simulink model "Pruefungsaufgabe_15"  (R2017b)
settings: Solver=ode45  StartTime=0.0  StopTime=5  FixedStep=0.001  MaxStep=1e-3  RelTol=1e-3  EnableMultiTasking=on
values from neighbouring files (symbols this model uses):
  CR = 2    [Pruefungsaufgabe_15_Konstanten.m]
  JRED = m1*R^2/(Ue^2*WGrad)    (= 0.000444444444444)    [Pruefungsaufgabe_15_Konstanten.m]
  KM = 38.4E-3    (= 0.0384)    [Pruefungsaufgabe_10_Konstanten.m]    (also in Pruefungsaufgabe_13_Konstanten.m = 0.05; Pruefungsaufgabe_15_Konstanten.m = 0.05)
  R = 0.02    [Pruefungsaufgabe_15_Konstanten.m]
  RA = 4.99    [Pruefungsaufgabe_10_Konstanten.m]    (also in Pruefungsaufgabe_13_Konstanten.m = 0.6; Pruefungsaufgabe_15_Konstanten.m = 5)
  Ue = 2    [Pruefungsaufgabe_15_Konstanten.m]
  WGrad = 0.9    [Pruefungsaufgabe_15_Konstanten.m]
undefined symbols (not defined in the file or in its folder): sigbuilder_block
libraries: simulink x2
settings Model: Creator=jbaur  LastModifiedBy=jbaur
settings DataIOCC: ExternalInput=X1  SaveFormat=StructureWithTime  InspectSignalLogs=on  SignalLoggingName=sigsOut
settings OptimizationCC: DefaultParameterBehavior=Inlined  InlineInvariantSignals=on  BufferReuse=off  ExpressionDepthLimit=2147483647  InitFltsAndDblsToZero=on  LifeSpan=inf
settings DebuggingCC: SaveWithParameterizedLinksMsg=none  SignalResolutionControl=TryResolveAllWithWarning  MultiTaskDSMMsg=warning  MultiTaskCondExecSysMsg=none  StateNameClashWarn=warning  InitInArrayFormatMsg=none  SFUnexpectedBacktrackingDiag=warning  SFNoUnconditionalDefaultTransitionDiag=warning  SFExecutionAtInitializationDiag=none
settings HardwareCC: ProdBitPerPointer=32  ProdBitPerSizeT=32  ProdBitPerPtrDiffT=32  ProdLargestAtomicFloat=None  ProdIntDivRoundTo=Undefined  ProdEndianess=Unspecified  ProdWordSize=32  ProdHWDeviceType=32-bit Generic  TargetBitPerPointer=64  TargetBitPerSizeT=64  TargetBitPerPtrDiffT=64  TargetLongLongMode=on  TargetIntDivRoundTo=Zero  TargetEndianess=LittleEndian  TargetWordSize=64  TargetHWDeviceType=MATLAB Host  ProdEqTarget=off
settings ModelReferenceCC: PropagateSignalLabelsOutOfModel=off
settings CodeAppCC: StateflowObjectComments=on
settings GRTTargetCC: TargetFcnLib=ansi_tfl_tmw.mat  TargetLangStandard=C89/C90 (ANSI)  ModelReferenceCompliant=off  GeneratePreprocessorConditionals=Disable all  CombineOutputUpdateFcns=off  MatFileLogging=off  GRTInterface=on
settings ConfigComp: CovMetricSettings=dw  CovHtmlReporting=on  CovSaveCumulativeToWorkspaceVar=on  CovSaveSingleToWorkspaceVar=on  CovExternalEMLEnable=off  CovSFcnEnable=off

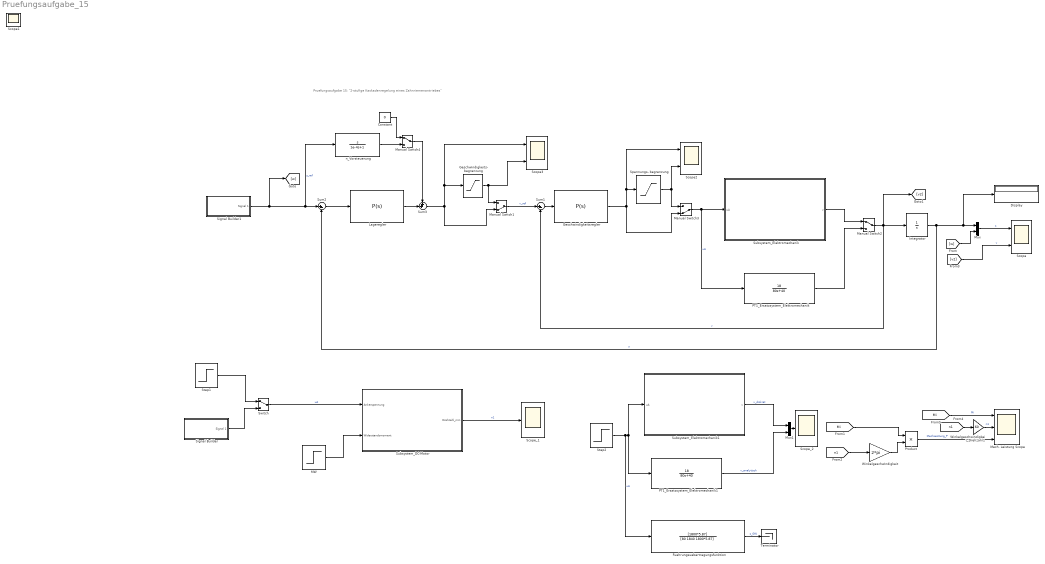
== system Pruefungsaufgabe_15 ==
  note: Pruefungsaufgabe 15: "2-stufige Kaskadenregelung eines Zahnriemenantriebes"
  Constant : Constant  Value=0
  Display : Display
  Fuehrungsuebertragungsfunktion : TransferFcn  Numerator=[1800*5.87]  Denominator=[80 1840 1800*5.87]
  Geschwindigkeits- begrenzung : Saturate  UpperLimit=4.77  LowerLimit=-4.77
  Geschwindigkeitsregler : simulink/Continuous/PID Controller  Controller=P  TimeDomain=Continuous-time  SampleTime=-1  IntegratorMethod=Forward Euler  FilterMethod=Forward Euler  Form=Parallel  UseFilter=on  ControllerParametersSource=internal  P=100  I=1000  D=0  N=1000  InitialConditionSource=internal  InitialConditionForIntegrator=0  InitialConditionForFilter=0  ExternalReset=none  LimitOutput=off  UpperSaturationLimit=24  LowerSaturationLimit=-24  LinearizeAsGain=off  AntiWindupMode=clamping  Kb=1000  TrackingMode=off  Kt=1  PParamMin=[]  PParamMax=[]  IParamMin=[]  IParamMax=[]  DParamMin=[]  DParamMax=[]  NParamMin=[]  NParamMax=[]  KbParamMin=[]  KbParamMax=[]  KtParamMin=[]  KtParamMax=[]  POutMin=[]  POutMax=[]  IOutMin=[]  IOutMax=[]  DOutMin=[]  DOutMax=[]  NOutMin=[]  NOutMax=[]  KbOutMin=[]  KbOutMax=[]  KtOutMin=[]  KtOutMax=[]  IntegratorOutMin=[]  IntegratorOutMax=[]  FilterOutMin=[]  FilterOutMax=[]  SumOutMin=[]  SumOutMax=[]  SumI1OutMin=[]  SumI1OutMax=[]  SumI2OutMin=[]  SumI2OutMax=[]  SumI3OutMin=[]  SumI3OutMax=[]  SumDOutMin=[]  SumDOutMax=[]  SaturationOutMin=[]  SaturationOutMax=[]  IntegratorContinuousStateAttributes=''  IntegratorStateMustResolveToSignalObject=off  IntegratorRTWStateStorageClass=Auto  FilterContinuousStateAttributes=''  FilterStateMustResolveToSignalObject=off  FilterRTWStateStorageClass=Auto  DifferentiatorICPrevScaledInput=0  DifferentiatorOutMin=[]  DifferentiatorOutMax=[]  InitialConditionSetting=State (most efficient)  FilterDiffOutCoefMin=[]  FilterDiffOutCoefMax=[]  SumDenOutMin=[]  SumDenOutMax=[]  SumNumOutMin=[]  SumNumOutMax=[]  ReciprocalOutMin=[]  ReciprocalOutMax=[]  DivideOutMin=[]  DivideOutMax=[]  TunerSelectOption=Transfer Function Based (PID Tuner App)
  Integrator : Integrator
  Lageregler : simulink/Continuous/PID Controller  Controller=P  TimeDomain=Continuous-time  SampleTime=-1  IntegratorMethod=Forward Euler  FilterMethod=Forward Euler  Form=Parallel  UseFilter=on  ControllerParametersSource=internal  P=5.87  I=2096.01243911413  D=0  N=100  InitialConditionSource=internal  InitialConditionForIntegrator=0  InitialConditionForFilter=0  ExternalReset=none  LimitOutput=off  UpperSaturationLimit=99  LowerSaturationLimit=-99  LinearizeAsGain=off  AntiWindupMode=none  Kb=1  TrackingMode=off  Kt=1  PParamMin=[]  PParamMax=[]  IParamMin=[]  IParamMax=[]  DParamMin=[]  DParamMax=[]  NParamMin=[]  NParamMax=[]  KbParamMin=[]  KbParamMax=[]  KtParamMin=[]  KtParamMax=[]  POutMin=[]  POutMax=[]  IOutMin=[]  IOutMax=[]  DOutMin=[]  DOutMax=[]  NOutMin=[]  NOutMax=[]  KbOutMin=[]  KbOutMax=[]  KtOutMin=[]  KtOutMax=[]  IntegratorOutMin=[]  IntegratorOutMax=[]  FilterOutMin=[]  FilterOutMax=[]  SumOutMin=[]  SumOutMax=[]  SumI1OutMin=[]  SumI1OutMax=[]  SumI2OutMin=[]  SumI2OutMax=[]  SumI3OutMin=[]  SumI3OutMax=[]  SumDOutMin=[]  SumDOutMax=[]  SaturationOutMin=[]  SaturationOutMax=[]  IntegratorContinuousStateAttributes=''  IntegratorStateMustResolveToSignalObject=off  IntegratorRTWStateStorageClass=Auto  FilterContinuousStateAttributes=''  FilterStateMustResolveToSignalObject=off  FilterRTWStateStorageClass=Auto  DifferentiatorICPrevScaledInput=0  DifferentiatorOutMin=[]  DifferentiatorOutMax=[]  InitialConditionSetting=State (most efficient)  FilterDiffOutCoefMin=[]  FilterDiffOutCoefMax=[]  SumDenOutMin=[]  SumDenOutMax=[]  SumNumOutMin=[]  SumNumOutMax=[]  ReciprocalOutMin=[]  ReciprocalOutMax=[]  DivideOutMin=[]  DivideOutMax=[]  TunerSelectOption=Transfer Function Based (PID Tuner App)
  MW : Step  Time=0  After=0.03  SampleTime=0
  Manual Switch1 : ManualSwitch  CurrentSetting=0
  Manual Switch2 : ManualSwitch
  Manual Switch3 : ManualSwitch  CurrentSetting=0
  Manual Switch4 : ManualSwitch
  Mech. Leistung Scope : Scope  NumInputPorts=3
  Mux : Mux  Inputs=2
  Mux1 : Mux  Inputs=2
  PT1_Ersatzsystem_Elektromechanik : TransferFcn  Numerator=[18]  Denominator=[80 40]
  PT1_Ersatzsystem_Elektromechanik1 : TransferFcn  Numerator=[18]  Denominator=[80 40]
  Product : Product  RndMeth=Zero
  Scope : Scope  NumInputPorts=2
  Scope2 : Scope  NumInputPorts=2
  Scope3 : Scope  NumInputPorts=2
  Scope_1 : Scope
  Scope_2 : Scope
  Signal Builder : Subsystem  Tag=STV Subsys  LoadFcn=sigbuilder_block('load');  StartFcn=sigbuilder_block('start');  StopFcn=sigbuilder_block('stop');  ClipboardFcn=sigbuilder_block('clipboard');  mask(Sigbuilder block){tuvar=[0:10]}
      mask help: Simulink:masks:SigbuilderBlock_MD
      mask init:
      | if ~strcmp(get_param(bdroot(gcbh),'SimulationStatus'),'stopped') tuvar = sigbuilder_block('maskInit'); end
      settings: CopyFcn=sigbuilder_block('copy');  DeleteFcn=sigbuilder_block('delete');  ModelCloseFcn=sigbuilder_block('modelClose');  PreSaveFcn=sigbuilder_block('preSave');  PauseFcn=sigbuilder_block('pause');  ContinueFcn=sigbuilder_block('continue');  NameChangeFcn=sigbuilder_block('namechange');  OpenFcn=sigbuilder_block('open',[437.25 199.5 550.5 399.75 ]);  CloseFcn=sigbuilder_block('close');
      mask Display: plot(0, 0, 100, 100,[2, 2, 32, 32, 2], [68, 8, 8, 68, 68],[32, 2], [38, 38], [32, 19, 2],[53, 60, 44], [32, 17, 17, 2],[16, 16, 31, 31]);txt = getActiveGroup(gcbh);text(2, 100, txt,'verticalAlignment', 'top');
  Signal Builder1 : Subsystem  Tag=STV Subsys  LoadFcn=sigbuilder_block('load');  StartFcn=sigbuilder_block('start');  StopFcn=sigbuilder_block('stop');  ClipboardFcn=sigbuilder_block('clipboard');  mask(Sigbuilder block){tuvar=[0:10]}
      mask help: Simulink:masks:SigbuilderBlock_MD
      mask init:
      | if ~strcmp(get_param(bdroot(gcbh),'SimulationStatus'),'stopped') tuvar = sigbuilder_block('maskInit'); end
      settings: CopyFcn=sigbuilder_block('copy');  DeleteFcn=sigbuilder_block('delete');  ModelCloseFcn=sigbuilder_block('modelClose');  PreSaveFcn=sigbuilder_block('preSave');  PauseFcn=sigbuilder_block('pause');  ContinueFcn=sigbuilder_block('continue');  NameChangeFcn=sigbuilder_block('namechange');  OpenFcn=sigbuilder_block('open',[437.25 199.5 550.5 399.75 ]);  CloseFcn=sigbuilder_block('close');
      mask Display: plot(0, 0, 100, 100,[2, 2, 32, 32, 2], [68, 8, 8, 68, 68],[32, 2], [38, 38], [32, 19, 2],[53, 60, 44], [32, 17, 17, 2],[16, 16, 31, 31]);txt = getActiveGroup(gcbh);text(2, 100, txt,'verticalAlignment', 'top');
  Spannungs- begrenzung : Saturate  UpperLimit=24  LowerLimit=-24
  Step1 : Step  Time=0  After=24  SampleTime=0
  Step2 : Step  Time=0  After=115  SampleTime=0
  Subsystem_DC-Motor : Subsystem
  Subsystem_Elektromechanik : Subsystem
  Subsystem_Elektromechanik1 : Subsystem
  Sum1 : Sum  Inputs=|+-  SaturateOnIntegerOverflow=on
  Sum2 : Sum  Inputs=|+-  SaturateOnIntegerOverflow=on
  Sum3 : Sum  Inputs=++|  SaturateOnIntegerOverflow=on
  Switch : ManualSwitch
  Terminator : Terminator
  Winkelgeschwindigkeit : Gain  Gain=2*pi
  Winkelgeschwindigkeit_Drehzahl1 : Gain  Gain=60
  n_Vorsteuerung : TransferFcn  Numerator=[1 0]  Denominator=[1e-4 1]
  Scope1 : Scope
  wires:
  Geschwindigkeitsregler/1 -> Manual Switch3/2, Scope2/1, Spannungs- begrenzung/1
  Spannungs- begrenzung/1 -> Manual Switch3/1, Scope2/2
  Manual Switch3/1 -> PT1_Ersatzsystem_Elektromechanik/1, Subsystem_Elektromechanik/1(uA)  "uA"
  Sum1/1 -> Geschwindigkeitsregler/1
  Sum2/1 -> Lageregler/1
  Manual Switch1/1 -> Sum1/1  "v_ref"
  Geschwindigkeits- begrenzung/1 -> Scope3/2, Manual Switch1/1
  [w] -> Mux/2
  [Mi] -> Product/1
  [n1] -> Winkelgeschwindigkeit/1
  Winkelgeschwindigkeit/1 -> Product/2
  Integrator/1 -> Display/1, Mux/1, Sum2/2  "s"
  Mux/1 -> Scope/1  "s"
  [v2] -> Scope/2  "v"
  Manual Switch2/1 -> Sum1/2, Integrator/1, [v2]  "v"
  PT1_Ersatzsystem_Elektromechanik/1 -> Manual Switch2/2
  Subsystem_Elektromechanik/1(v) -> Manual Switch2/1
  Signal Builder1/1(Signal 1) -> n_Vorsteuerung/1, Sum2/1, [w]  "s_ref"
  Subsystem_DC-Motor/1(Drehzahl_min) -> Scope_1/1  "n1"
  Step1/1 -> Switch/1
  Signal Builder/1(Signal 1) -> Switch/2
  Switch/1 -> Subsystem_DC-Motor/1(Ankerspannung)  "uA"
  MW/1 -> Subsystem_DC-Motor/2(Widerstandsmoment)
  Product/1 -> Mech. Leistung Scope/3  "MechLeistung_P"
  [n1] -> Winkelgeschwindigkeit_Drehzahl1/1
  [Mi] -> Mech. Leistung Scope/1  "Mi"
  Winkelgeschwindigkeit_Drehzahl1/1 -> Mech. Leistung Scope/2  "n1"
  Step2/1 -> Fuehrungsuebertragungsfunktion/1, Subsystem_Elektromechanik1/1(uA), PT1_Ersatzsystem_Elektromechanik1/1  "uA"
  Subsystem_Elektromechanik1/1(v) -> Mux1/1  "v_diskret"
  PT1_Ersatzsystem_Elektromechanik1/1 -> Mux1/2  "v_analytisch"
  Lageregler/1 -> Sum3/2
  Sum3/1 -> Manual Switch1/2, Scope3/1, Geschwindigkeits- begrenzung/1
  n_Vorsteuerung/1 -> Manual Switch4/2
  Manual Switch4/1 -> Sum3/1
  Constant/1 -> Manual Switch4/1
  Mux1/1 -> Scope_2/1
  Fuehrungsuebertragungsfunktion/1 -> Terminator/1  "s_GW"

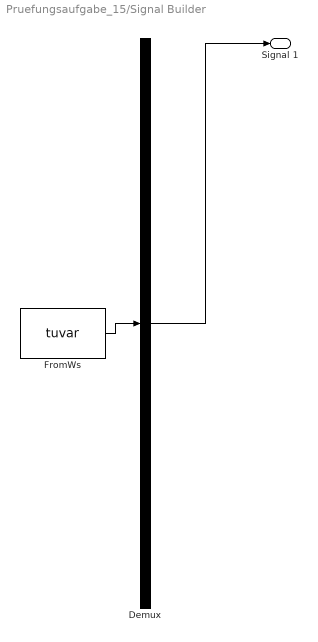
== system Pruefungsaufgabe_15/Signal Builder ==
  Demux : Demux  Tag=STV Demux  Outputs=1
  FromWs : FromWorkspace  Tag=STV FromWs  VariableName=tuvar  SampleTime=0
      SigBuilderData=|
      | common.afterFinalStr = 'Extrapolate'
      | common.sampleTime = 0
      | dataSet.timeRange = [0 10]
      | dataSet.name = 'Group 1'
      | sbobj.Groups.Name = 'Group 1'
      | sbobj.Groups.Signals.Name = 'Signal 1'
      | sbobj.Groups.Signals.XData = [0 1 1 2 2 10]
      | sbobj.Groups.Signals.YData = [0 0 24 24 0 0]
  Signal 1 : Outport  Tag=STV Outport
  wires:
  Demux/1 -> Signal 1/1
  FromWs/1 -> Demux/1

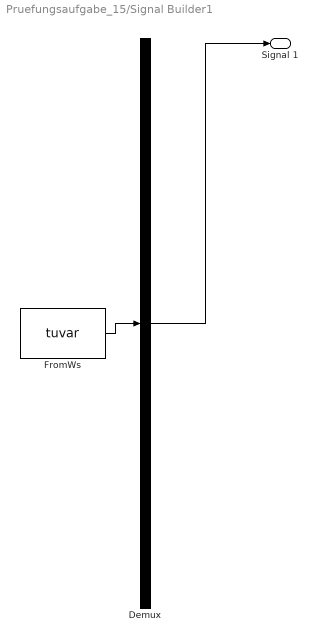
== system Pruefungsaufgabe_15/Signal Builder1 ==
  Demux : Demux  Tag=STV Demux  Outputs=1
  FromWs : FromWorkspace  Tag=STV FromWs  VariableName=tuvar  SampleTime=0
      SigBuilderData=|
      | common.afterFinalStr = 'Extrapolate'
      | common.sampleTime = 0
      | dataSet.timeRange = [0 10]
      | dataSet.name = 'Group 1'
      | sbobj.Groups.Name = 'Group 1'
      | sbobj.Groups.Signals.Name = 'Signal 1'
      | sbobj.Groups.Signals.XData = [0 1 2 10]
      | sbobj.Groups.Signals.YData = [0 0 1 1]
  Signal 1 : Outport  Tag=STV Outport
  wires:
  Demux/1 -> Signal 1/1
  FromWs/1 -> Demux/1

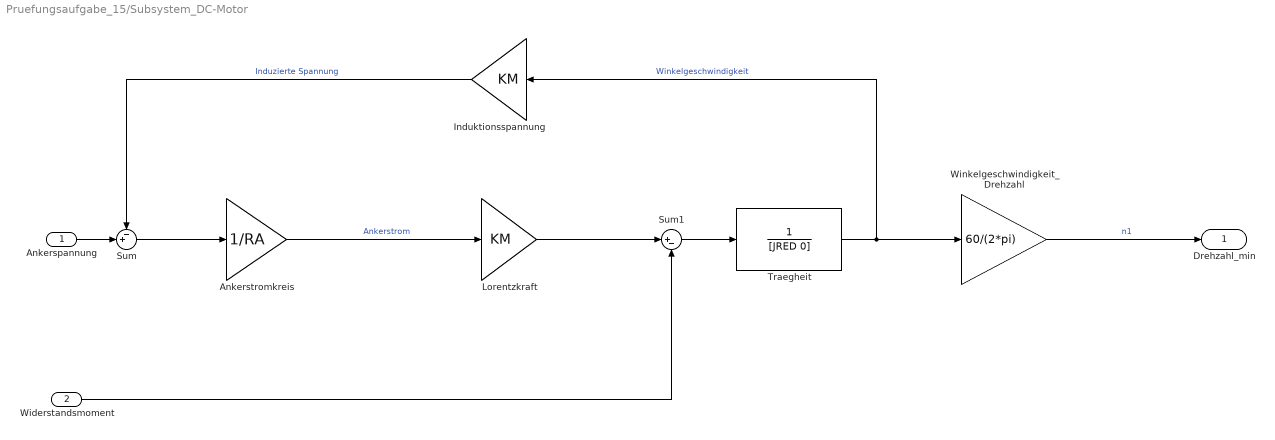
== system Pruefungsaufgabe_15/Subsystem_DC-Motor ==
  Ankerspannung : Inport
  Widerstandsmoment : Inport  Port=2
  Ankerstromkreis : Gain  Gain=1/RA
  Induktionsspannung : Gain  Gain=KM
  Lorentzkraft : Gain  Gain=KM
  Sum : Sum  Inputs=-+|
  Sum1 : Sum  Inputs=|+-
  Traegheit : TransferFcn  Denominator=[JRED 0]
  Winkelgeschwindigkeit_Drehzahl : Gain  Gain=60/(2*pi)
  Drehzahl_min : Outport
  wires:
  Winkelgeschwindigkeit_Drehzahl/1 -> Drehzahl_min/1  "n1"
  Ankerspannung/1 -> Sum/2
  Sum/1 -> Ankerstromkreis/1
  Traegheit/1 -> Induktionsspannung/1, Winkelgeschwindigkeit_Drehzahl/1  "Winkelgeschwindigkeit"
  Lorentzkraft/1 -> Sum1/1
  Sum1/1 -> Traegheit/1
  Ankerstromkreis/1 -> Lorentzkraft/1  "Ankerstrom"
  Induktionsspannung/1 -> Sum/1  "Induzierte Spannung"
  Widerstandsmoment/1 -> Sum1/2

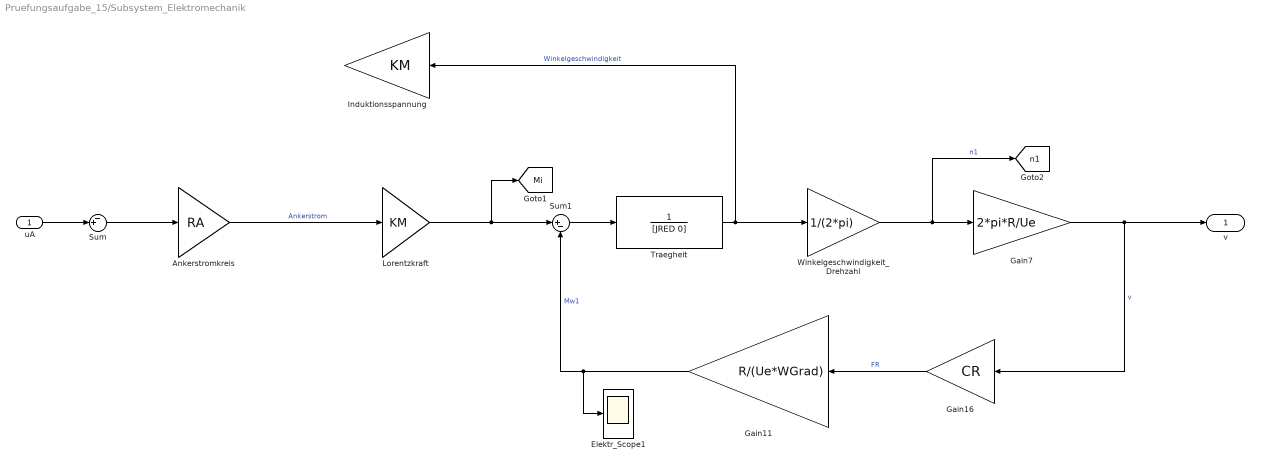
== system Pruefungsaufgabe_15/Subsystem_Elektromechanik ==
  uA : Inport
  Ankerstromkreis : Gain  Gain=RA
  Elektr_Scope1 : Scope
  Gain11 : Gain  Gain=R/(Ue*WGrad)
  Gain16 : Gain  Gain=CR
  Gain7 : Gain  Gain=2*pi*R/Ue
  Induktionsspannung : Gain  Gain=KM
  Lorentzkraft : Gain  Gain=KM
  Sum : Sum  Inputs=-+|
  Sum1 : Sum  Inputs=|+-
  Traegheit : TransferFcn  Denominator=[JRED 0]
  Winkelgeschwindigkeit_Drehzahl : Gain  Gain=1/(2*pi)
  v : Outport
  tag scope: Mi=global, n1=global
  wires:
  Winkelgeschwindigkeit_Drehzahl/1 -> [n1], Gain7/1  "n1"
  Sum/1 -> Ankerstromkreis/1
  Traegheit/1 -> Induktionsspannung/1, Winkelgeschwindigkeit_Drehzahl/1  "Winkelgeschwindigkeit"
  Lorentzkraft/1 -> [Mi], Sum1/1
  Sum1/1 -> Traegheit/1
  Ankerstromkreis/1 -> Lorentzkraft/1  "Ankerstrom"
  Gain7/1 -> Gain16/1, v/1  "v"
  Gain11/1 -> Elektr_Scope1/1, Sum1/2  "Mw1"
  Gain16/1 -> Gain11/1  "FR"
  uA/1 -> Sum/2

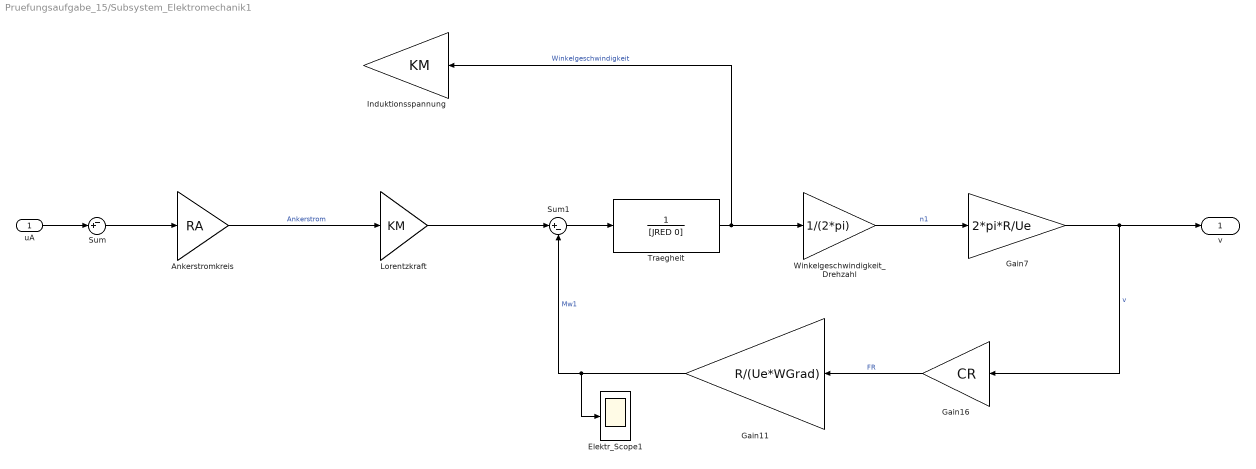
== system Pruefungsaufgabe_15/Subsystem_Elektromechanik1 ==
  uA : Inport
  Ankerstromkreis : Gain  Gain=RA
  Elektr_Scope1 : Scope
  Gain11 : Gain  Gain=R/(Ue*WGrad)
  Gain16 : Gain  Gain=CR
  Gain7 : Gain  Gain=2*pi*R/Ue
  Induktionsspannung : Gain  Gain=KM
  Lorentzkraft : Gain  Gain=KM
  Sum : Sum  Inputs=-+|
  Sum1 : Sum  Inputs=|+-
  Traegheit : TransferFcn  Denominator=[JRED 0]
  Winkelgeschwindigkeit_Drehzahl : Gain  Gain=1/(2*pi)
  v : Outport
  wires:
  Winkelgeschwindigkeit_Drehzahl/1 -> Gain7/1  "n1"
  Sum/1 -> Ankerstromkreis/1
  Traegheit/1 -> Induktionsspannung/1, Winkelgeschwindigkeit_Drehzahl/1  "Winkelgeschwindigkeit"
  Lorentzkraft/1 -> Sum1/1
  Sum1/1 -> Traegheit/1
  Ankerstromkreis/1 -> Lorentzkraft/1  "Ankerstrom"
  Gain7/1 -> Gain16/1, v/1  "v"
  Gain11/1 -> Elektr_Scope1/1, Sum1/2  "Mw1"
  Gain16/1 -> Gain11/1  "FR"
  uA/1 -> Sum/2
